simulink model "LEGO_NXT_M1V4_Closed_Loop_DC_Motor_Position_Control"  (R2017b)
settings: Solver=FixedStepDiscrete  StartTime=0.0  StopTime=45  FixedStep=.003  RelTol=1e-3  EnableMultiTasking=on
values from neighbouring files (symbols this model uses):
  G = (1/(Ra+La*s))*Kt*(1/(J*s^2+b*s))    [EE_A472_HW1.m]    (also in MiniLab04_Motor_Skeleton.m = -inv(C*inv(A-B*Kdisk)*B); linearization_lecture.m)
  Kdisk = place(motorDiscrete.A,motorDiscrete.B,pDisc)    [MiniLab04_Motor_Skeleton.m]
  L = place(motorDiscrete.A',motorDiscrete.C',pDiscObs)'    [MiniLab04_Motor_Skeleton.m]    (also in MiniLab05_Motor_Skeleton.m)
  motorDiscrete = c2d(motor_ss,Ts)    [MiniLab04_Motor_Skeleton.m]    (also in MiniLab05_Motor_Skeleton.m)
libraries: MinSegLibrary_M1V4 x2
settings Model: SimulationMode=external  ExtModeTrigDuration=2  Creator=malcoj2  LastModifiedBy=Erik
settings DataIOCC: LimitDataPoints=on  SaveFormat=Array
settings OptimizationCC: PassReuseOutputArgsThreshold=0  MaxStackSize=64
settings DebuggingCC: UnderspecifiedInitializationDetection=Classic  MergeDetectMultiDrivingBlocksExec=none  ParameterTunabilityLossMsg=error  StateNameClashWarn=warning  SFUnexpectedBacktrackingDiag=warning  SFNoUnconditionalDefaultTransitionDiag=warning  SFExecutionAtInitializationDiag=none
settings HardwareCC: ProdBitPerInt=16  ProdBitPerPointer=16  ProdBitPerSizeT=16  ProdBitPerPtrDiffT=16  ProdLargestAtomicFloat=None  ProdWordSize=8  ProdHWDeviceType=Atmel->AVR  UseEmbeddedCoderFeatures=off
settings ModelReferenceCC: PropagateSignalLabelsOutOfModel=off
settings SFSimCC: MATLABDynamicMemAlloc=off
settings RTWCC: SystemTargetFile=ert.tlc  HardwareBoard=Arduino Mega 2560  TLCOptions=-aInlineSetEventsForThisBaseRateFcn=TLC_FALSE -aSuppressMultiTaskScheduler=TLC_FALSE -aRateBasedStepFcn=1  TemplateMakefile=ert_default_tmf  GenerateReport=on  RTWVerbose=off  Toolchain=Arduino AVR  BuildConfiguration=Faster Runs  LaunchReport=on
settings CodeAppCC: ForceParamTrailComments=on  OperatorAnnotations=on  StateflowObjectComments=on  MATLABSourceComments=on
settings ERTTargetCC: ERTCustomFileBanners=off  SupportContinuousTime=on  SupportNonInlinedSFcns=on  RemoveResetFunc=off  SupportVariableSizeSignals=on  ModelStepFunctionPrototypeControlCompliant=off
settings ConfigComp: CovMetricSettings=dw  CovHtmlReporting=on  CovSaveCumulativeToWorkspaceVar=on  CovSaveSingleToWorkspaceVar=on  CovExternalEMLEnable=off

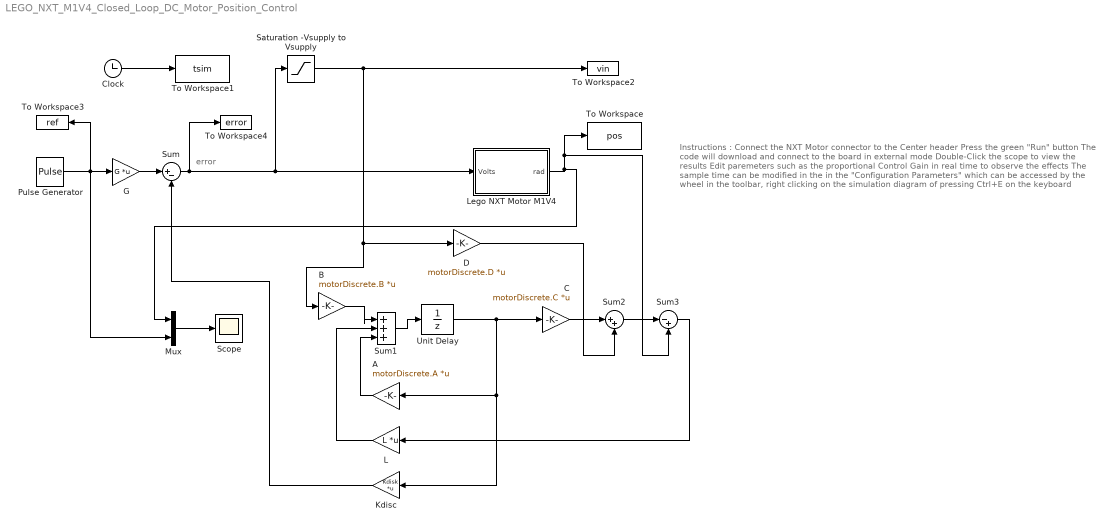
== system LEGO_NXT_M1V4_Closed_Loop_DC_Motor_Position_Control ==
  note: error
  note: Instructions :
      | Connect the NXT Motor connector to the Center header
      | Press the green "Run" button
      | The code will download and connect to the board in external mode
      | Double-Click the scope to view the results
      | Edit paremeters such as the proportional Control Gain in real time to observe the effects
      |
      | The sample time can be modified in the in the "Configuration Parameters" which can be accessed by the wheel in the toolbar, right clicking on the simulation diagram of pressing Ctrl+E on the keyboard
  A : Gain  Gain=motorDiscrete.A  Multiplication=Matrix(K*u)
  B : Gain  Gain=motorDiscrete.B  Multiplication=Matrix(K*u)
  C : Gain  Gain=motorDiscrete.C  Multiplication=Matrix(K*u)
  Clock : Clock
  D : Gain  Gain=motorDiscrete.D  Multiplication=Matrix(K*u)
  G : Gain  Gain=G  Multiplication=Matrix(K*u)
  Kdisc : Gain  Gain=Kdisk  Multiplication=Matrix(K*u)
  L : Gain  Gain=L  Multiplication=Matrix(K*u)
  Lego NXT Motor M1V4 : Subsystem
  Mux : Mux  Inputs=2
  Pulse Generator : DiscretePulseGenerator  PulseType=Time based  Amplitude=90*pi/180  Period=3  PulseWidth=50
  Saturation -Vsupply to Vsupply : Saturate  UpperLimit=3.25  LowerLimit=-3.25  OutDataTypeStr=single
  Scope : Scope
  Sum : Sum  Inputs=|+-
  Sum1 : Sum  Inputs=|+++
  Sum2 : Sum  Inputs=|++
  Sum3 : Sum  Inputs=|-+
  To Workspace : ToWorkspace  VariableName=pos  SampleTime=-1
  To Workspace1 : ToWorkspace  VariableName=tsim  SampleTime=-1
  To Workspace2 : ToWorkspace  VariableName=vin  SampleTime=-1
  To Workspace3 : ToWorkspace  VariableName=ref  SampleTime=-1
  To Workspace4 : ToWorkspace  VariableName=error  SampleTime=-1
  Unit Delay : UnitDelay  SampleTime=-1
  wires:
  Clock/1 -> To Workspace1/1
  Pulse Generator/1 -> G/1, Mux/2, To Workspace3/1
  Lego NXT Motor M1V4/1(rad) -> Mux/1, Sum3/2, To Workspace/1
  Sum/1 -> Lego NXT Motor M1V4/1(Volts), Saturation -Vsupply to Vsupply/1, To Workspace4/1
  Saturation -Vsupply to Vsupply/1 -> B/1, D/1, To Workspace2/1
  B/1 -> Sum1/1
  Sum1/1 -> Unit Delay/1
  Unit Delay/1 -> Kdisc/1, A/1, C/1
  A/1 -> Sum1/3
  L/1 -> Sum1/2
  Kdisc/1 -> Sum/2
  Sum2/1 -> Sum3/1
  Sum3/1 -> L/1
  C/1 -> Sum2/1
  D/1 -> Sum2/2
  Mux/1 -> Scope/1
  G/1 -> Sum/1

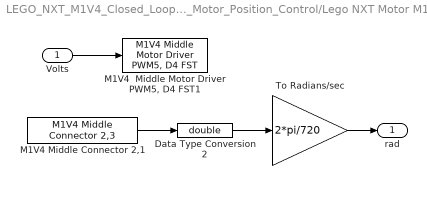
== system LEGO_NXT_M1V4_Closed_Loop_DC_Motor_Position_Control/Lego NXT Motor M1V4 ==
  Volts : Inport
  Data Type Conversion2 : DataTypeConversion  OutDataTypeStr=double
  "M1V4  Middle Motor Driver PWM5, D4 FST1" : MinSegLibrary_M1V4/M1V4  Middle Motor Driver PWM5, D4 FST  Vsupply=3.25
      settings: SourceProductName=Rensselaer Arduino Support Package
  M1V4 Middle Connector 2,1 : MinSegLibrary_M1V4/M1V4 Middle Connector 2,3  Encoder=0  PinA=3  PinB=2  PWMFSelect=3  PWMTimer=-1
      settings: SourceProductName=Rensselaer Arduino Support Package
  To Radians/sec : Gain  Gain=2*pi/720
  rad : Outport
  wires:
  To Radians/sec/1 -> rad/1
  M1V4 Middle Connector 2,1/1 -> Data Type Conversion2/1
  Volts/1 -> "M1V4  Middle Motor Driver PWM5, D4 FST1"/1
  Data Type Conversion2/1 -> To Radians/sec/1
